simulink model "softLanding_sim"  (R2024b)
settings: Solver=VariableStepAuto  StartTime=0.0  StopTime=200  RelTol=1e-3
settings Model: Creator=JEEVESH  LastModifiedBy=JEEVESH

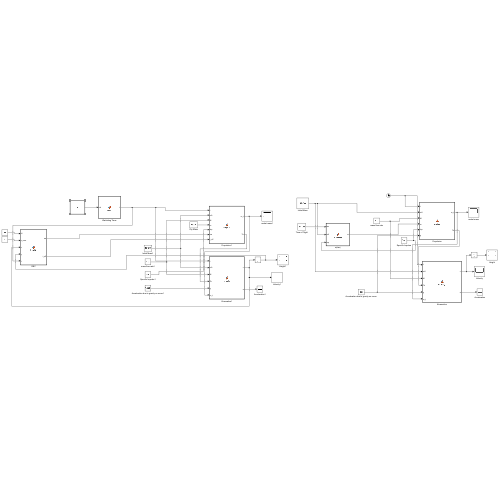
[thumbnail: Simulink's stored preview of the top-level diagram]
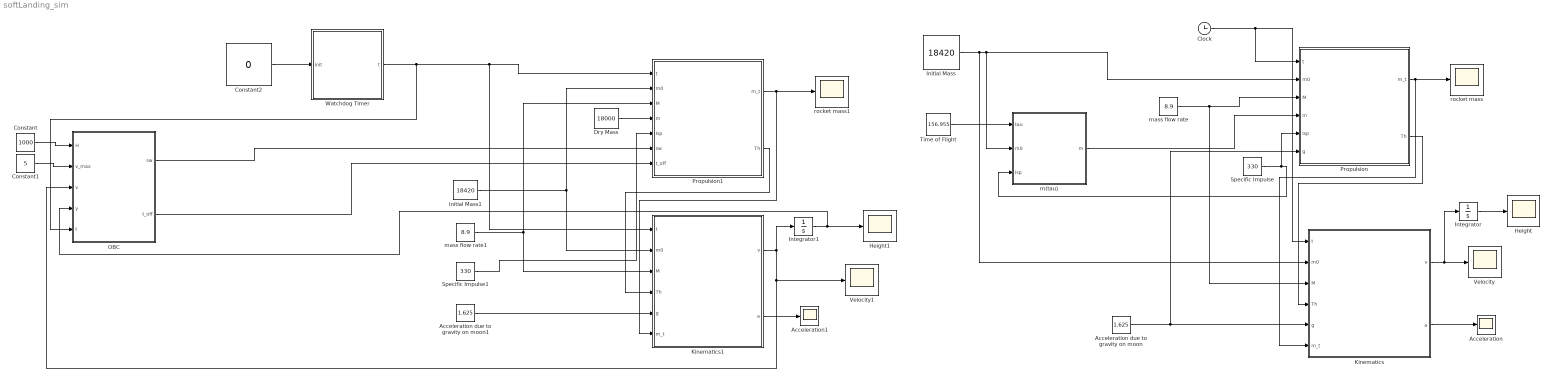
== system softLanding_sim ==
  Acceleration : Scope
  Acceleration due to gravity on moon : Constant  Value=1.625
  Acceleration due to gravity on moon1 : Constant  Value=1.625
  Acceleration1 : Scope
  Clock : Clock
  Constant : Constant  Value=1000
  Constant1 : Constant  Value=5
  Constant2 : Constant  Value=0
  Dry Mass : Constant  Value=18000
  Height : Scope
  Height1 : Scope
  Initial Mass : Constant  Value=18420
  Initial Mass1 : Constant  Value=18420
  Integrator : Integrator
  Integrator1 : Integrator
  Kinematics : MATLAB Function  TreatAsAtomicUnit=on
  Kinematics1 : MATLAB Function  TreatAsAtomicUnit=on
  OBC : MATLAB Function  TreatAsAtomicUnit=on
  Propulsion : MATLAB Function  TreatAsAtomicUnit=on
  Propulsion1 : MATLAB Function  TreatAsAtomicUnit=on
  Specific Impulse : Constant  Value=330
  Specific Impulse1 : Constant  Value=330
  Time of Flight : Constant  Value=156.955
  Velocity : Scope
  Velocity1 : Scope
  Watchdog Timer : MATLAB Function  TreatAsAtomicUnit=on
  m(tau) : MATLAB Function  TreatAsAtomicUnit=on
  mass flow rate : Constant  Value=8.9
  mass flow rate1 : Constant  Value=8.9
  rocket mass : Scope
  rocket mass1 : Scope
  wires:
  Clock/1 -> Kinematics/1(t), Propulsion/1(t)
  Propulsion/1(m_t) -> Kinematics/6(m_t), rocket mass/1
  Initial Mass/1 -> Propulsion/2(m0), m(tau)/2(m0), Kinematics/2(m0)
  Kinematics/1(v) -> Integrator/1, Velocity/1
  mass flow rate/1 -> Kinematics/3(M), Propulsion/3(M)
  Acceleration due to gravity on moon/1 -> Propulsion/6(g), Kinematics/5(g)
  Kinematics/2(a) -> Acceleration/1
  Integrator/1 -> Height/1
  Specific Impulse/1 -> m(tau)/3(Isp), Propulsion/5(Isp)
  Propulsion/2(Th) -> Kinematics/4(Th)
  Time of Flight/1 -> m(tau)/1(tau)
  m(tau)/1(m) -> Propulsion/4(m)
  Initial Mass1/1 -> Kinematics1/2(m0), Propulsion1/2(m0)
  mass flow rate1/1 -> Kinematics1/3(M), Propulsion1/3(M)
  Specific Impulse1/1 -> Propulsion1/5(Isp)
  Acceleration due to gravity on moon1/1 -> Kinematics1/5(g)
  Propulsion1/1(m_t) -> rocket mass1/1, Kinematics1/6(m_t)
  Propulsion1/2(Th) -> Kinematics1/4(Th)
  Kinematics1/1(v) -> Velocity1/1, OBC/3(v), Integrator1/1
  Constant1/1 -> OBC/2(v_max)
  Constant/1 -> OBC/1(H)
  Integrator1/1 -> Height1/1, OBC/4(y)
  OBC/1(sw) -> Propulsion1/6(sw)
  OBC/2(t_off) -> Propulsion1/7(t_off)
  Dry Mass/1 -> Propulsion1/4(m)
  Kinematics1/2(a) -> Acceleration1/1
  Constant2/1 -> Watchdog Timer/1(init)
  Watchdog Timer/1(t) -> OBC/5(t), Kinematics1/1(t), Propulsion1/1(t)

== matlab function softLanding_sim/Kinematics1 ==
  data: t input; v output; m0 input; M input; Th input; g input; m_t input; a output
function [v,a] = velocity(t, m0, M, Th, g, m_t)
% Calculates the velocity after engine starts

v_calc = g * t - (Th/M) * log(m0/m_t);
a_calc = g - Th/m_t;

% If velocity drops below zero, keep it at zero and acceleration at g
v = max(0, v_calc);
if v ~= 0
    a = a_calc;
else
    a = g;

end

== matlab function softLanding_sim/m(tau) ==
  data: tau input; m output; m0 input; Isp input
function m = finalMass(tau,m0,Isp)

m = m0 * exp(-tau/Isp);

end

== matlab function softLanding_sim/Kinematics ==
  data: t input; v output; m0 input; M input; Th input; g input; m_t input; a output
function [v,a] = velocity(t, m0, M, Th, g, m_t)
% Calculates the velocity after engine starts

v_calc = g * t - (Th/M) * log(m0/m_t);
a_calc = g - Th/m_t;

% If velocity drops below zero, keep it at zero and acceleration at g
v = max(0, v_calc);
if v ~= 0
    a = a_calc;
else
    a = g;

end

== matlab function softLanding_sim/Propulsion ==
  data: t input; m_t output; m0 input; M input; m input; Isp input; g input; Th output
function [m_t,Th] = engine(t, m0, M,m,Isp,g)
% Calculates the mass of a rocket at time t
% Inputs:
%   t  - time 
%   v - velocity at time t
%   m0 - initial mass 
%   M  - mass flow rate 
% Output:
%   m_t  - mass at time t

m_cal = m0 - M * t;
m_t = max(m_cal,m);

Th = Isp*M*9.8;

end

== matlab function softLanding_sim/Propulsion1 ==
  data: t input; m_t output; m0 input; M input; m input; Isp input; Th output; sw input; t_off input
function [m_t, Th] = engine(t, m0, M, m, Isp, sw, t_off)
    
Th = Isp * M * 9.8;

if sw == true
    m_t = m0 - M * t;
else
   m_t = m0 - m * t_off;
end

== matlab function softLanding_sim/OBC ==
  data: H input; sw output; t_off output; v_max input; v input; y input; t input
function [sw, t_off] = throttle(H,v_max,v,y,t)

sw = false;
t_prev = 0;
while y ~= H
    if v == v_max
        sw = true;
        t_prev = t;
    else if v == 0
        sw = false;
        t_off = t_prev;
    else
        sw = false;
        t_off = t_prev;
    end
end

end

== matlab function softLanding_sim/Watchdog Timer ==
  data: init input; t output
function t = time(init)

t = init + 0.001;

end
